simulink model "ECM_2021"  (R2021a)
settings: Solver=FixedStepAuto  StartTime=0.0  StopTime=params.Tend  FixedStep=params.Ts  RelTol=1e-3
model workspace (MAT data in the model file):
  p = [3.8 3.8 3.8 3.8 3.8 3.8]
values from neighbouring files (symbols this model uses):
  params = obs_default.init.params    [first_guess.m]    (also in params_battery_tushar.m = first_guess(params,params_sim))
undefined symbols (not defined in the file or in its folder): obs_s, sigbuilder_block
libraries: simulink x2, autolibrcnetworksystem x1
settings Model: Creator=tkddesai  LastModifiedBy=fedeoli

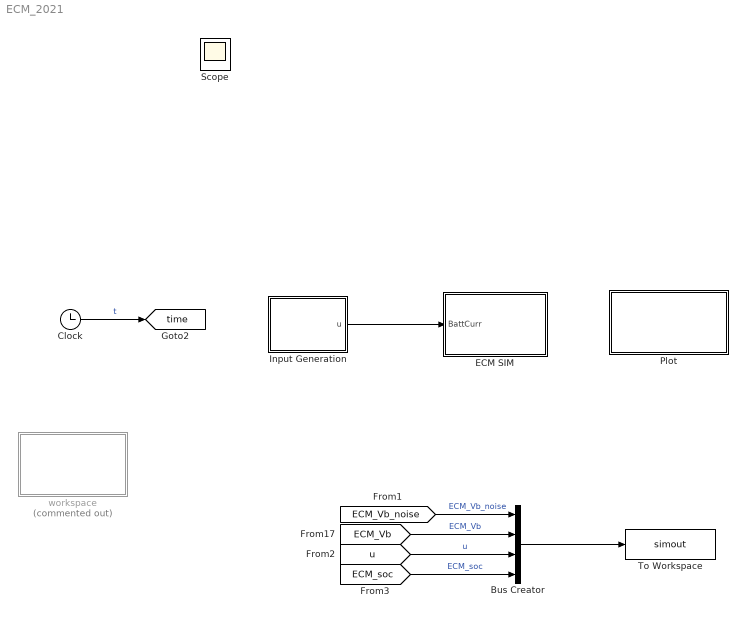
== system ECM_2021 ==
  Bus Creator : BusCreator  Inputs=4
  Clock : Clock
  ECM SIM : Subsystem
  Input Generation : Subsystem
  Plot : Subsystem
  To Workspace : ToWorkspace  VariableName=simout  SaveFormat=Timeseries  SampleTime=-1
  workspace : Subsystem  Commented=on
  Scope : Scope
  tag scope: time=global
  wires:
  Input Generation/1(u) -> ECM SIM/1(BattCurr)
  Clock/1 -> [time]  "t"
  [ECM_Vb_noise] -> Bus Creator/1  "ECM_Vb_noise"
  [ECM_Vb] -> Bus Creator/2  "ECM_Vb"
  [u] -> Bus Creator/3  "u"
  [ECM_soc] -> Bus Creator/4  "ECM_soc"
  Bus Creator/1 -> To Workspace/1

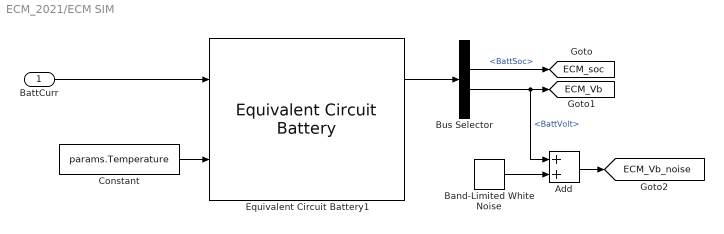
== system ECM_2021/ECM SIM ==
  BattCurr : Inport
  Add : Sum
  Band-Limited White Noise : simulink/Sources/Band-Limited White Noise  Cov=params.NoisePwr  Ts=params.Ts  seed=[23341]
  Bus Selector : BusSelector  OutputSignals=BattCurr,BattSoc,BattVolt,BattPwr
  Constant : Constant  Value=params.Temperature
  Equivalent Circuit Battery1 : autolibrcnetworksystem/Equivalent Circuit Battery  CapacityCtrl=Parameter  OutputVlt=Unfiltered  NumRC=1  Em=[params.input_soc, params.input_OCV_nominal]  R0=[params.input_soc, params.input_R0_nominal]  SOC_BP=params.input_soc  Temperature_BP=[293.15 313.15]  BattCap=[params.C_n_h_nominal params.C_n_h_nominal]  BattCapInit=params.C_n_h_nominal  InitialCapVoltage=params.X.val(2,1)  Tc=1/1000  Vinit=4.193  R1=[params.input_soc, params.input_R1_nominal]  C1=[params.input_soc, params.input_C1_nominal]  R2=|  C2=|  R3=|  C3=|  R4=|  C4=|  R5=|  C5=|  Vu=Inf  Vl=-Inf  RefBlkName='autolibrcnetworksystem/Equivalent Circuit Battery'
      R2=|
      | [0.010342 0.0012244;
      | 0.0067316 0.0011396;
      | 0.0051156 0.0012661;
      | 0.0043447 0.0012265;
      | 0.0038826 0.0011163;
      | 0.0034226 0.0009968;
      | 0.003346 0.0011458;
      | 0.0033222 0.001345;
      | 0.0033201 0.0013091;
      | 0.0032886 0.0010986;
      | 0.0028114 0.0010309]
      C2=|
      | [2287.7 11897;
      | 6122 24515;
      | 18460 42098;
      | 20975 44453;
      | 15254 33098;
      | 10440 24492;
      | 13903 32975;
      | 16694 40007;
      | 15784 35937;
      | 12165 26430;
      | 9118 24795]
      R3=|
      | [0.010342 0.0012244;
      | 0.0067316 0.0011396;
      | 0.0051156 0.0012661;
      | 0.0043447 0.0012265;
      | 0.0038826 0.0011163;
      | 0.0034226 0.0009968;
      | 0.003346 0.0011458;
      | 0.0033222 0.001345;
      | 0.0033201 0.0013091;
      | 0.0032886 0.0010986;
      | 0.0028114 0.0010309]
      C3=|
      | [2287.7 11897;
      | 6122 24515;
      | 18460 42098;
      | 20975 44453;
      | 15254 33098;
      | 10440 24492;
      | 13903 32975;
      | 16694 40007;
      | 15784 35937;
      | 12165 26430;
      | 9118 24795]
      R4=|
      | [0.010342 0.0012244;
      | 0.0067316 0.0011396;
      | 0.0051156 0.0012661;
      | 0.0043447 0.0012265;
      | 0.0038826 0.0011163;
      | 0.0034226 0.0009968;
      | 0.003346 0.0011458;
      | 0.0033222 0.001345;
      | 0.0033201 0.0013091;
      | 0.0032886 0.0010986;
      | 0.0028114 0.0010309]
      C4=|
      | [2287.7 11897;
      | 6122 24515;
      | 18460 42098;
      | 20975 44453;
      | 15254 33098;
      | 10440 24492;
      | 13903 32975;
      | 16694 40007;
      | 15784 35937;
      | 12165 26430;
      | 9118 24795]
      R5=|
      | [0.010342 0.0012244;
      | 0.0067316 0.0011396;
      | 0.0051156 0.0012661;
      | 0.0043447 0.0012265;
      | 0.0038826 0.0011163;
      | 0.0034226 0.0009968;
      | 0.003346 0.0011458;
      | 0.0033222 0.001345;
      | 0.0033201 0.0013091;
      | 0.0032886 0.0010986;
      | 0.0028114 0.0010309]
      C5=|
      | [2287.7 11897;
      | 6122 24515;
      | 18460 42098;
      | 20975 44453;
      | 15254 33098;
      | 10440 24492;
      | 13903 32975;
      | 16694 40007;
      | 15784 35937;
      | 12165 26430;
      | 9118 24795]
      settings: SourceProductBaseCode=PW
  tag scope: ECM_Vb=global, ECM_Vb_noise=global, ECM_soc=global
  wires:
  Bus Selector/3 -> Add/1, [ECM_Vb]  "<BattVolt>"
  Bus Selector/2 -> [ECM_soc]  "<BattSoc>"
  Equivalent Circuit Battery1/1 -> Bus Selector/1
  Constant/1 -> Equivalent Circuit Battery1/2
  BattCurr/1 -> Equivalent Circuit Battery1/1
  Band-Limited White Noise/1 -> Add/2
  Add/1 -> [ECM_Vb_noise]

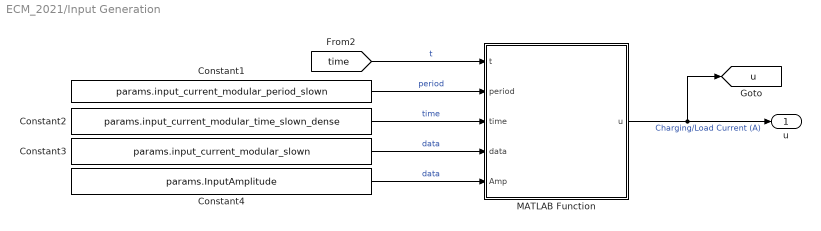
== system ECM_2021/Input Generation ==
  Constant1 : Constant  Value=params.input_current_modular_period_slown
  Constant2 : Constant  Value=params.input_current_modular_time_slown_dense
  Constant3 : Constant  Value=params.input_current_modular_slown
  Constant4 : Constant  Value=params.InputAmplitude
  MATLAB Function : MATLAB Function  TreatAsAtomicUnit=on
  u : Outport
  tag scope: u=global
  wires:
  MATLAB Function/1(u) -> [u], u/1  "Charging/Load Current (A)"
  [time] -> MATLAB Function/1(t)  "t"
  Constant1/1 -> MATLAB Function/2(period)  "period"
  Constant2/1 -> MATLAB Function/3(time)  "time"
  Constant3/1 -> MATLAB Function/4(data)  "data"
  Constant4/1 -> MATLAB Function/5(Amp)  "data"

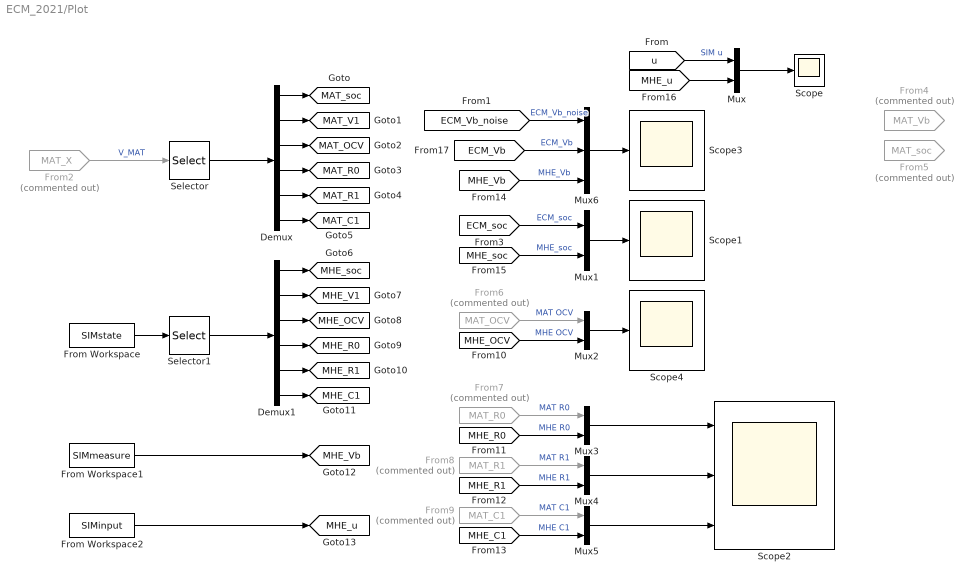
== system ECM_2021/Plot ==
  Demux : Demux  Outputs=6
  Demux1 : Demux  Outputs=6
  From Workspace : FromWorkspace  VariableName=SIMstate
  From Workspace1 : FromWorkspace  VariableName=SIMmeasure
  From Workspace2 : FromWorkspace  VariableName=SIMinput
  From2 : From  Commented=on  GotoTag=MAT_X  TagVisibility=global
  From4 : From  Commented=on  GotoTag=MAT_Vb  TagVisibility=global
  From5 : From  Commented=on  GotoTag=MAT_soc  TagVisibility=global
  From6 : From  Commented=on  GotoTag=MAT_OCV  TagVisibility=global
  From7 : From  Commented=on  GotoTag=MAT_R0  TagVisibility=global
  From8 : From  Commented=on  GotoTag=MAT_R1  TagVisibility=global
  From9 : From  Commented=on  GotoTag=MAT_C1  TagVisibility=global
  Mux{,1..5} (6 alike) : Mux  Inputs=2
  Mux6 : Mux  Inputs=3
  Scope{,1,3..4} (4 alike) : Scope
  Scope2 : Scope  NumInputPorts=3
  Selector : Selector  InputPortWidth=obs_s{1}.setup.dim_state  IndexOptions=Index vector (dialog)  Indices=[1 2 3 4 5 6]  OutputSizes=1
  Selector1 : Selector  InputPortWidth=obs_s{1}.setup.dim_state  IndexOptions=Index vector (dialog)  Indices=[1 2 3 4 5 6]  OutputSizes=1
  tag scope: MAT_C1=global, MAT_OCV=global, MAT_R0=global, MAT_R1=global, MAT_V1=global, MAT_soc=global, MHE_C1=global, MHE_OCV=global, MHE_R0=global, MHE_R1=global, MHE_V1=global, MHE_Vb=global, MHE_soc=global, MHE_u=global
  wires:
  [ECM_Vb_noise] -> Mux6/1  "ECM_Vb_noise"
  From2/1 -> Selector/1  "V_MAT"
  [ECM_soc] -> Mux1/1  "ECM_soc"
  Selector/1 -> Demux/1
  Demux/1 -> [MAT_soc]
  Demux/2 -> [MAT_V1]
  Mux1/1 -> Scope1/1
  Mux6/1 -> Scope3/1
  Demux/3 -> [MAT_OCV]
  Demux/4 -> [MAT_R0]
  Demux/5 -> [MAT_R1]
  Demux/6 -> [MAT_C1]
  Mux4/1 -> Scope2/2
  Mux5/1 -> Scope2/3
  From Workspace/1 -> Selector1/1
  Demux1/6 -> [MHE_C1]
  Demux1/5 -> [MHE_R1]
  Demux1/4 -> [MHE_R0]
  Demux1/3 -> [MHE_OCV]
  Demux1/2 -> [MHE_V1]
  Demux1/1 -> [MHE_soc]
  Selector1/1 -> Demux1/1
  From6/1 -> Mux2/1  "MAT OCV"
  From7/1 -> Mux3/1  "MAT R0"
  From8/1 -> Mux4/1  "MAT R1"
  From9/1 -> Mux5/1  "MAT C1"
  [MHE_OCV] -> Mux2/2  "MHE OCV"
  [MHE_R0] -> Mux3/2  "MHE R0"
  [MHE_R1] -> Mux4/2  "MHE R1"
  [MHE_C1] -> Mux5/2  "MHE C1"
  From Workspace1/1 -> [MHE_Vb]
  [MHE_soc] -> Mux1/2  "MHE_soc"
  Mux/1 -> Scope/1
  [u] -> Mux/1  "SIM u"
  From Workspace2/1 -> [MHE_u]
  [MHE_u] -> Mux/2
  [MHE_Vb] -> Mux6/3  "MHE_Vb"
  [ECM_Vb] -> Mux6/2  "ECM_Vb"
  Mux2/1 -> Scope4/1
  Mux3/1 -> Scope2/1

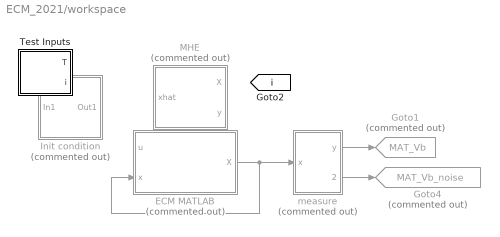
== system ECM_2021/workspace ==
  ECM MATLAB : Subsystem  Commented=on
  Goto1 : Goto  Commented=on  GotoTag=MAT_Vb  TagVisibility=global
  Goto4 : Goto  Commented=on  GotoTag=MAT_Vb_noise  TagVisibility=global
  Init condition : Subsystem  Commented=on
  MHE : Subsystem  Commented=on
  Test Inputs : Subsystem
  measure : Subsystem  Commented=on
  tag scope: i=global
  wires:
  measure/1(y) -> Goto1/1
  measure/2(y_noise) -> Goto4/1
  ECM MATLAB/1(X) -> ECM MATLAB/2(x), measure/1(x)

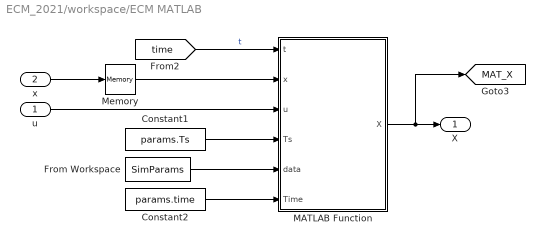
== system ECM_2021/workspace/ECM MATLAB ==
  u : Inport
  x : Inport  Port=2
  Constant1 : Constant  Value=params.Ts
  Constant2 : Constant  Value=params.time
  From Workspace : FromWorkspace  VariableName=SimParams
  MATLAB Function : MATLAB Function  TreatAsAtomicUnit=on
  Memory : Memory  InitialCondition=obs_s{1}.init.X_est.val(:,1)
  X : Outport
  tag scope: MAT_X=global
  wires:
  x/1 -> Memory/1
  From Workspace/1 -> MATLAB Function/5(data)
  MATLAB Function/1(X) -> [MAT_X], X/1
  Constant1/1 -> MATLAB Function/4(Ts)
  u/1 -> MATLAB Function/3(u)
  [time] -> MATLAB Function/1(t)  "t"
  Memory/1 -> MATLAB Function/2(x)
  Constant2/1 -> MATLAB Function/6(Time)

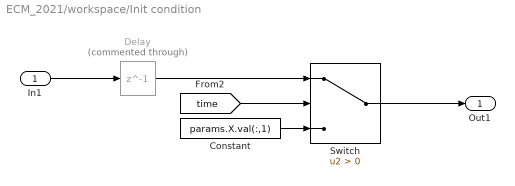
== system ECM_2021/workspace/Init condition ==
  In1 : Inport
  Constant : Constant  Value=params.X.val(:,1)
  Delay : Delay  Commented=through  DelayLength=1  InitialCondition=0
  Switch : Switch  Criteria=u2 > Threshold
  Out1 : Outport
  wires:
  Constant/1 -> Switch/3
  [time] -> Switch/2
  Switch/1 -> Out1/1
  In1/1 -> Delay/1
  Delay/1 -> Switch/1

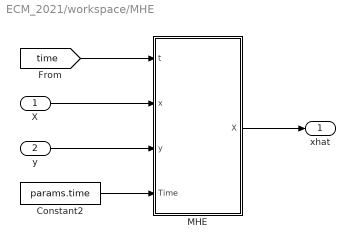
== system ECM_2021/workspace/MHE ==
  X : Inport
  y : Inport  Port=2
  Constant2 : Constant  Value=params.time
  MHE : MATLAB Function  TreatAsAtomicUnit=on
  xhat : Outport
  wires:
  MHE/1(X) -> xhat/1
  X/1 -> MHE/2(x)
  y/1 -> MHE/3(y)
  [time] -> MHE/1(t)
  Constant2/1 -> MHE/4(Time)

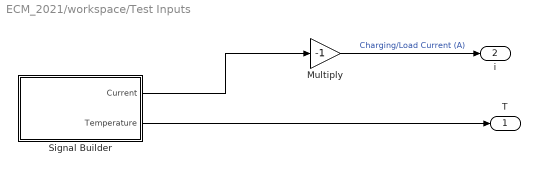
== system ECM_2021/workspace/Test Inputs ==
  Multiply : Gain  Gain=-1
  Signal Builder : Subsystem  Tag=STV Subsys  LoadFcn=sigbuilder_block('load');  StartFcn=sigbuilder_block('start');  StopFcn=sigbuilder_block('stop');  ClipboardFcn=sigbuilder_block('clipboard');  mask(Sigbuilder block){tuvar=[0:10]}
      mask help: Simulink:masks:SigbuilderBlock_MD
      mask init:
      | if ~strcmp(get_param(bdroot(gcbh),'SimulationStatus'),'stopped') tuvar = sigbuilder_block('maskInit'); end
      settings: CopyFcn=sigbuilder_block('copy');  DeleteFcn=sigbuilder_block('delete');  ModelCloseFcn=sigbuilder_block('modelClose');  PreSaveFcn=sigbuilder_block('preSave');  PauseFcn=sigbuilder_block('pause');  ContinueFcn=sigbuilder_block('continue');  NameChangeFcn=sigbuilder_block('namechange');  OpenFcn=sigbuilder_block('open',[292.5 181.5 1147.5 535.5 ]);  CloseFcn=sigbuilder_block('close');
      mask Display: plot(0, 0, 100, 100,[2, 2, 32, 32, 2], [68, 8, 8, 68, 68],[32, 2], [38, 38], [32, 19, 2],[53, 60, 44], [32, 17, 17, 2],[16, 16, 31, 31]);txt = getActiveGroup(gcbh);text(2, 100, txt,'verticalAlignment', 'top');
  T : Outport  VectorParamsAs1DForOutWhenUnconnected=off
  i : Outport  Port=2  VectorParamsAs1DForOutWhenUnconnected=off
  wires:
  Signal Builder/1(Current) -> Multiply/1
  Multiply/1 -> i/1  "Charging/Load Current (A)"
  Signal Builder/2(Temperature) -> T/1

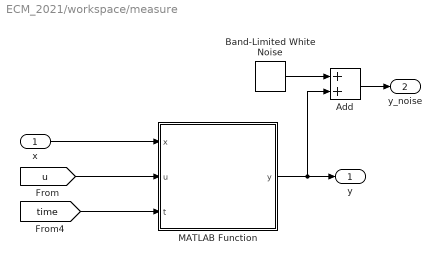
== system ECM_2021/workspace/measure ==
  x : Inport
  Add : Sum
  Band-Limited White Noise : simulink/Sources/Band-Limited White Noise  Cov=[0.1]  Ts=params.Ts  seed=[23341]
  MATLAB Function : MATLAB Function  TreatAsAtomicUnit=on
  y : Outport
  y_noise : Outport  Port=2
  wires:
  [u] -> MATLAB Function/2(u)
  MATLAB Function/1(y) -> Add/2, y/1
  x/1 -> MATLAB Function/1(x)
  [time] -> MATLAB Function/3(t)
  Band-Limited White Noise/1 -> Add/1
  Add/1 -> y_noise/1

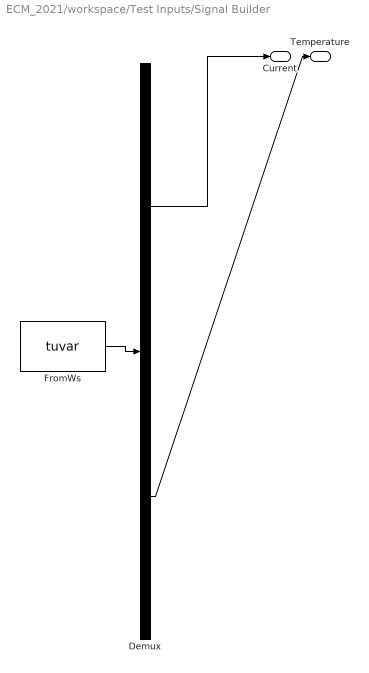
== system ECM_2021/workspace/Test Inputs/Signal Builder ==
  Demux : Demux  Tag=STV Demux  Outputs=2
      settings: DisplayOption=none
  FromWs : FromWorkspace  Tag=STV FromWs  VariableName=tuvar
      SigBuilderData=|
      | common.afterFinalStr = 'Extrapolate'
      | common.sampleTime = 0
      | dataSet.timeRange = [1 6698]
      | dataSet.name = 'Sheet1'
      | sbobj.Name = 'Signal Builder'
      | sbobj.Groups.Name = 'Sheet1'
      | sbobj.Groups.Signals(1).Name = 'Current'
      | sbobj.Groups.Signals(1).XData = [1 2 3 4 5 6 7 8 9 10 11 12 ... (6698 elements, 1x6698)]
      | sbobj.Groups.Signals(1).YData = [-1.9243103452e-05 -1.9243103452e-05 -1.9243103452e-05 -1.9243103452e-05 -1.9243103452e-05 -1.9243103452e-05 -1.9243103452e-05 -1.9243103452e-05 -1.9243103452e-05 -1.9243103452e-05 -1.9243103452e-05 -1.9243103452e-05 ... (6698 elements, 1x6698)]
      | sbobj.Groups.Signals(2).Name = 'Temperature'
      | sbobj.Groups.Signals(2).XData = [1 2 3 4 5 6 7 8 9 10 11 12 ... (6698 elements, 1x6698)]
      | sbobj.Groups.Signals(2).YData = [298.15 298.15 298.15 298.15 298.15 298.15 298.15 298.15 298.15 298.15 298.15 298.15 ... (6698 elements, 1x6698)]
      | sbobj.Groups.TimeRange = [1 6698]
  Current : Outport  Tag=STV Outport  VectorParamsAs1DForOutWhenUnconnected=off
  Temperature : Outport  Tag=STV Outport  Port=2
  wires:
  FromWs/1 -> Demux/1
  Demux/1 -> Current/1
  Demux/2 -> Temperature/1

== matlab function ECM_2021/workspace/ECM MATLAB/MATLAB Function ==
  data: t input; x input; u input; X output; Ts input; data input; Time input
function X = integrate(t,x,u,Ts,data,Time)

    % extrinsic fcn
    coder.extrinsic('wrapper_integrate');   

    % init out
    X = x(:,1);

    X = wrapper_integrate(t,x,u,Ts,data,Time);

end

== matlab function ECM_2021/Input Generation/MATLAB Function ==
  data: t input; u output; period input; time input; data input; Amp input
function u = input(t,period,time,data,Amp)   

    len = min(length(time),length(data));
    u = -Amp*interp1(time(1:len),data(1:len),mod(t,period),'previous');  

end

== matlab function ECM_2021/workspace/measure/MATLAB Function ==
  data: x input; u input; y output; t input
function y = measure(x,u,t)

    % coder
    coder.extrinsic('wrapper_measure');

    % init
    y = 0;
    % measure

    y = wrapper_measure(x,u,t);

end

== matlab function ECM_2021/workspace/MHE/MHE ==
  data: t input; X output; x input; y input; Time input
function X = observer(t,x,y,Time)

    % extrinsic fcn
    coder.extrinsic('wrapper_observer');   

    % init out
    X = x(:,1);

    % MHE
    X = wrapper_observer(t,x,y,Time,obs);
    
end
